simulink model "sim_aircraftGear"  (Simulink 7.4)
settings: Solver=ode45  StartTime=0.0  StopTime=10.0  MaxStep=0.005  RelTol=1e-3
PreLoadFcn:
  | setGlobalVariables();
undefined symbols (not defined in the file or in its folder): createExamplesPath, getInstallDir
libraries: EAsimulink x1
settings Model: Creator=fct  LastModifiedBy=fct
settings DataIOCC: SignalLoggingName=sigsOut
settings OptimizationCC: InitFltsAndDblsToZero=on
settings DebuggingCC: SaveWithParameterizedLinksMsg=none  SignalResolutionControl=TryResolveAllWithWarning  SolverPrmCheckMsg=none  MultiTaskDSMMsg=warning  MultiTaskCondExecSysMsg=none  StrictBusMsg=None
settings HardwareCC: TargetUnknown=on
settings RTWCC: IncludeERTFirstTime=on
settings GRTTargetCC: TargetFcnLib=ansi_tfl_tmw.mat

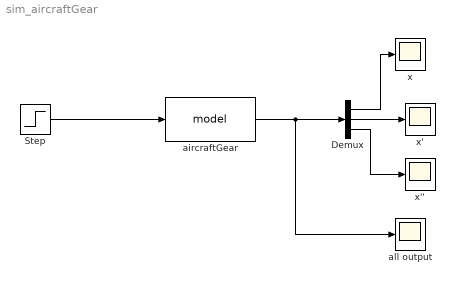
== system sim_aircraftGear ==
  Demux : Demux  Outputs=3
  Step : Step  Time=2  Before=2042.6  After=300  SampleTime=0
  aircraftGear : EAsimulink/model  modelFile=createExamplesPath('aircraft+gear', 'default', 'exp1')  installDir=getInstallDir()  inVars='m1'  outVars='x x'' x'''''  s_cint=0.01  e_cint=0.1
  all output : Scope
      settings: TimeRange=10  YMin=-100  YMax=200  SaveName=ScopeData2
  x : Scope
  x' : Scope
  x'' : Scope
      settings: SaveName=ScopeData3
  wires:
  Demux/1 -> x/1
  Demux/2 -> x'/1
  Demux/3 -> x''/1
  aircraftGear/1 -> Demux/1, all output/1
  Step/1 -> aircraftGear/1
